simulink model "cubli_XYZ_extensive_simulations"  (R2016a)
(part 8 of 9)

         -(11529215046068469760000*(173808361171031714041*cos(th3) - 97421867139278569472*sin(th3)))/(50688073959935957106266099682798465939237*cos(th2)),                                                      -(11529215046068469760000*(97421867139278569472*cos(th3) - 173808361171031714041*sin(th3)))/(50688073959935957106266099682798465939237*cos(th2)),                                                                        -(1123197656438253912603716965936891166720000*2^(1/2)*cos(th3 + pi/4))/(50688073959935957106266099682798465939237*cos(th2))
         - (1123197656438253912603716965936891166720000*cos(th3))/50688073959935957106266099682798465939237 - (2003873972745561633640040521298775900160000*sin(th3))/50688073959935957106266099682798465939237, - (2003873972745561633640040521298775900160000*cos(th3))/50688073959935957106266099682798465939237 - (1123197656438253912603716965936891166720000*sin(th3))/50688073959935957106266099682798465939237,                                                                                   -(1123197656438253912603716965936891166720000*2^(1/2)*sin(th3 + pi/4))/50688073959935957106266099682798465939237
         -(11529215046068469760000*(97421867139278569472*cos(th2) - 173808361171031714041*cos(th3)*sin(th2) + 97421867139278569472*sin(th2)*sin(th3)))/(50688073959935957106266099682798465939237*cos(th2)),    -(11529215046068469760000*(97421867139278569472*cos(th2) - 97421867139278569472*cos(th3)*sin(th2) + 173808361171031714041*sin(th2)*sin(th3)))/(50688073959935957106266099682798465939237*cos(th2)), -(11529215046068469760000*(173808361171031714041*cos(th2) - 97421867139278569472*cos(th3)*sin(th2) + 97421867139278569472*sin(th2)*sin(th3)))/(50688073959935957106266099682798465939237*cos(th2))
         3279361077300893534217161825852213947980628648106796253184/827891082019760530150909915741403671266755252589300489, 1123197656438253912603716965936891166720000/50688073959935957106266099682798465939237, 1123197656438253912603716965936891166720000/50688073959935957106266099682798465939237
         1123197656438253912603716965936891166720000/50688073959935957106266099682798465939237, 3279361077300893534217161825852213947980628648106796253184/827891082019760530150909915741403671266755252589300489, 1123197656438253912603716965936891166720000/50688073959935957106266099682798465939237
         1123197656438253912603716965936891166720000/50688073959935957106266099682798465939237, 1123197656438253912603716965936891166720000/50688073959935957106266099682798465939237, 3279361077300893534217161825852213947980628648106796253184/827891082019760530150909915741403671266755252589300489
        ];
    
    C = eye(9);

    % evaluate canonical form to avoid
    % failure in evaluation of lqr gain
    % due to non controllable unstable modes
    [Aalt, Balt, ~, T, ~] = ctrbf(A,B,C,10^-6);
    
    % evaluate LQR gain
    Q_lqr = T * Q * T.';
    [K, ~, ~] = lqr(Aalt(2:9,2:9),Balt(2:9,1:3),Q_lqr(2:9,2:9),R);
    K_lqr = [zeros(3,1), K] * T;
end

% control law
delta_x = state - state_eq;
u = - K_lqr *  delta_x ;

end
